simulink model "FULL_13_2_2019"  (R2024b)
settings: Solver=VariableStepAuto  StartTime=0.0  StopTime=10.0  RelTol=1e-3
settings Model: Creator=DT User  LastModifiedBy=DT User

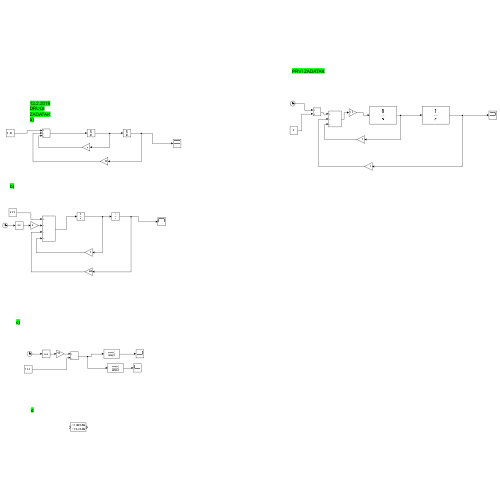
[thumbnail: Simulink's stored preview of the top-level diagram]
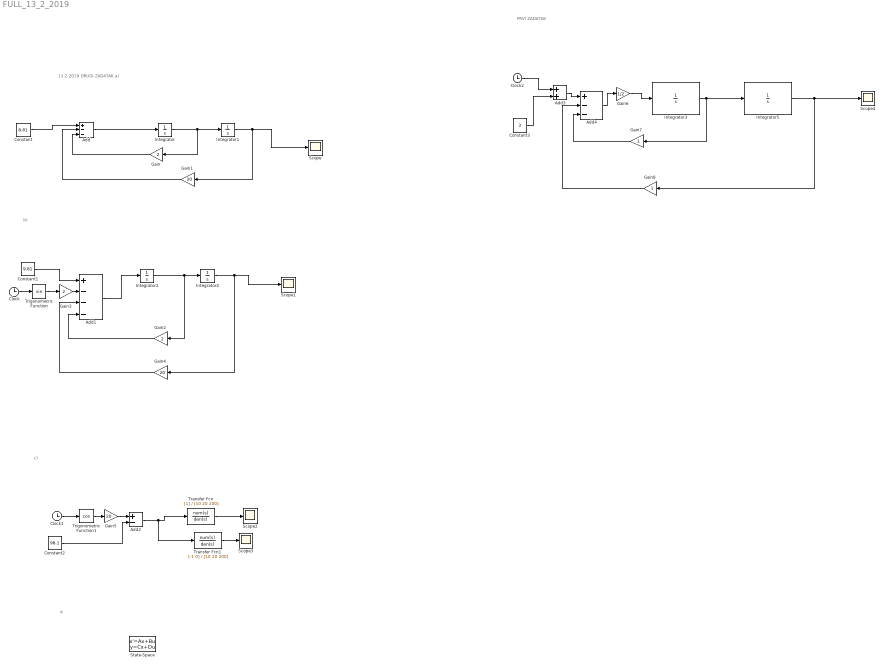
== system FULL_13_2_2019 ==
  note: PRVI ZADATAK
  note: d
  note: c)
  note: b)
  note: 13.2.2019
      | DRUGI ZADATAK
      | a)
  Add : Sum  Inputs=+--
  Add1 : Sum  Inputs=+---
  Add2 : Sum  Inputs=+-
  Add3 : Sum
  Add4 : Sum  Inputs=+--
  Clock : Clock
  Clock1 : Clock
  Clock2 : Clock
  Constant : Constant  Value=8.81
  Constant1 : Constant  Value=9.81
  Constant2 : Constant  Value=98.1
  Constant3 : Constant  Value=3
  Gain : Gain  Gain=2
  Gain1 : Gain  Gain=20
  Gain2 : Gain  Gain=2
  Gain3 : Gain  Gain=2
  Gain4 : Gain  Gain=20
  Gain5 : Gain  Gain=20
  Gain6 : Gain  Gain=1/2
  Gain7 : Gain
  Gain8 : Gain
  Integrator{,1..2,4} (4 alike) : Integrator
  Integrator3 : Integrator  InitialCondition=1
  Integrator5 : Integrator  InitialCondition=2
  Scope{,1..4} (5 alike) : Scope
  State-Space : StateSpace  InitialCondition=0
  Transfer Fcn : TransferFcn  Denominator=[10 20 200]
  Transfer Fcn1 : TransferFcn  Numerator=[-1 0]  Denominator=[10 20 200]
  Trigonometric Function : Trigonometry
  Trigonometric Function1 : Trigonometry  Operator=cos
  wires:
  Integrator/1 -> Gain/1, Integrator1/1
  Add/1 -> Integrator/1
  Integrator1/1 -> Gain1/1, Scope/1
  Constant/1 -> Add/1
  Gain/1 -> Add/3
  Gain1/1 -> Add/2
  Integrator2/1 -> Gain2/1, Integrator4/1
  Integrator4/1 -> Gain4/1, Scope1/1
  Clock/1 -> Trigonometric Function/1
  Trigonometric Function/1 -> Gain3/1
  Gain3/1 -> Add1/2
  Constant1/1 -> Add1/1
  Gain2/1 -> Add1/4
  Gain4/1 -> Add1/3
  Add1/1 -> Integrator2/1
  Clock1/1 -> Trigonometric Function1/1
  Trigonometric Function1/1 -> Gain5/1
  Transfer Fcn/1 -> Scope2/1
  Gain5/1 -> Add2/1
  Constant2/1 -> Add2/2
  Add2/1 -> Transfer Fcn1/1, Transfer Fcn/1
  Transfer Fcn1/1 -> Scope3/1
  Integrator5/1 -> Gain8/1, Scope4/1
  Integrator3/1 -> Gain7/1, Integrator5/1
  Gain6/1 -> Integrator3/1
  Clock2/1 -> Add3/1
  Constant3/1 -> Add3/2
  Add3/1 -> Add4/1
  Add4/1 -> Gain6/1
  Gain7/1 -> Add4/3
  Gain8/1 -> Add4/2
